simulink model "probe_tut1"  (Simulink 5.0)
settings: Solver=ode45  StartTime=0.0  StopTime=10.0  RelTol=1e-3
libraries: dspsigops x2, dspsrcs4 x1
settings Model: Creator=ckamachi  LastModifiedBy=ckamachi  BlockReductionOpt=off  BooleanDataType=off

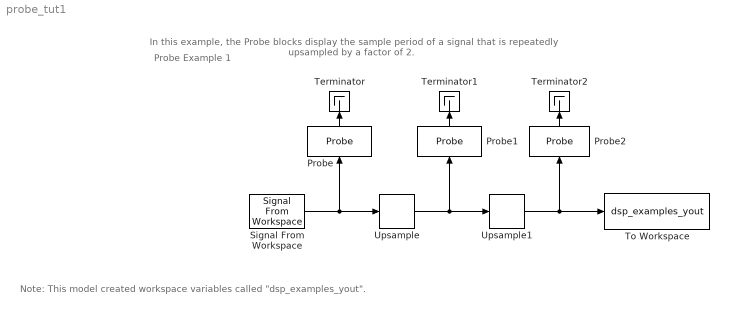
== system probe_tut1 ==
  note: Probe Example 1
  note: In this example, the Probe blocks display the sample period of a signal that is
      | repeatedly upsampled by a factor of 2.
  note: Note: This model created workspace variables called "dsp_examples_yout".
  Probe : Probe  Orientation=up  ProbeWidth=off  ProbeComplexSignal=off
  Probe1 : Probe  Orientation=up  ProbeWidth=off  ProbeComplexSignal=off
  Probe2 : Probe  Orientation=up  ProbeWidth=off  ProbeComplexSignal=off
  Signal From Workspace : dspsrcs4/Signal From Workspace  X=1:1000  Ts=1  nsamps=1  OutputAfterFinalValue=Setting to zero
  Terminator : Terminator
      settings: Orientation=up
  Terminator1 : Terminator
      settings: Orientation=up
  Terminator2 : Terminator
      settings: Orientation=up
  To Workspace : ToWorkspace  VariableName=dsp_examples_yout  SampleTime=-1  SaveFormat=Array
  Upsample : dspsigops/Upsample  N=2  phase=0  ic=0  mode=Maintain input frame size
  Upsample1 : dspsigops/Upsample  N=2  phase=0  ic=0  mode=Maintain input frame size
  wires:
  Signal From Workspace/1 -> Upsample/1, Probe/1
  Upsample/1 -> Upsample1/1, Probe1/1
  Upsample1/1 -> To Workspace/1, Probe2/1
  Probe/1 -> Terminator/1
  Probe1/1 -> Terminator1/1
  Probe2/1 -> Terminator2/1
